simulink model "simulation_main"  (R2025b)
settings: Solver=FixedStepAuto  StartTime=0.0  StopTime=40  RelTol=1e-3
StartFcn:
  | MaxMissedTicks = 99^100;
  | SampleTime = 0.01;
libraries: simulink x5, SignalEditorBlockLib x3
settings Model: Creator=labadmin  LastModifiedBy=David
settings HardwareCC: ProdBitPerLong=64.0  ProdHWDeviceType=Intel->x86-64 (Linux 64)
settings RTWCC: SystemTargetFile=sldrt.tlc  TemplateMakefile=sldrt.tmf  RTWCompilerOptimization=on  GPUComputeCapability=3.5  Description=Simulink Desktop Real-Time
settings CodeAppCC: MaxIdLength=95.0
settings SimulinkDesktopRealTimeCC: ExtModeTransport=0.0  ExtModeStaticAllocSize=1000000.0  TargetLibSuffix=_sldrt.a  TargetPreCompLibLocation=C:\Program Files\MATLAB\R2025b\toolbox\sldrt\lib\win64  MultiwordLength=2048.0  DynamicStringBufferSize=256.0  ParMdlRefBuildCompliant=on  PreserveMATLABNamespacesInGeneratedCode=on  SubcomponentCodeInterfacePackaging=Reusable function

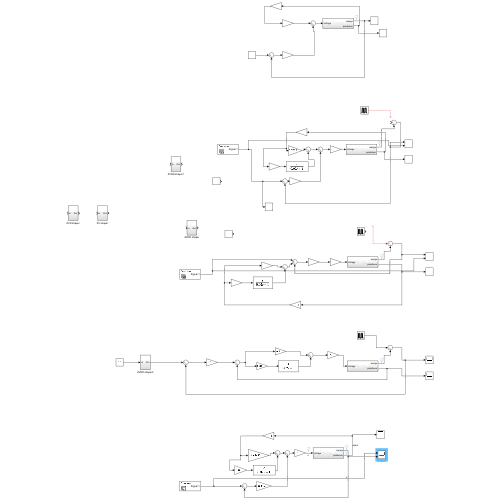
[thumbnail: Simulink's stored preview of the top-level diagram]
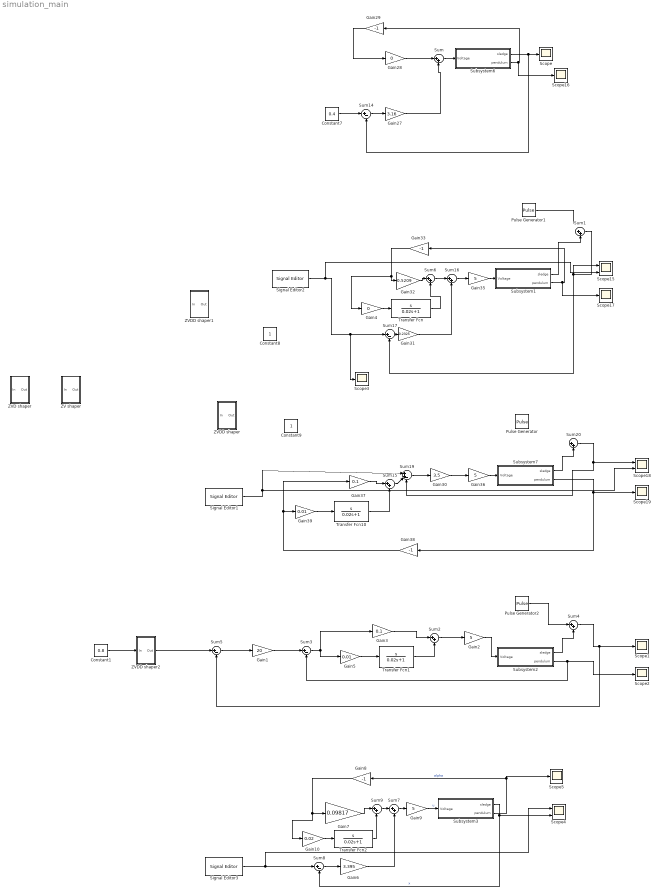
== system simulation_main ==
  Constant1 : Constant  Value=0.8
  Constant7 : Constant  Value=0.4
  Constant8 : Constant
  Constant9 : Constant
  Gain1 : Gain  Gain=20
  Gain10 : Gain  Gain=0.02
  Gain{2,9,35..36} (4 alike) : Gain  Gain=5
  Gain27 : Gain  Gain=3.16
  Gain28 : Gain  Gain=0
  Gain{8,29,33,38} (4 alike) : Gain  Gain=-1
  Gain3 : Gain  Gain=0.1
  Gain30 : Gain  Gain=3.5
  Gain31 : Gain  Gain=0.2325
  Gain32 : Gain  Gain=0.5209
  Gain37 : Gain  Gain=0.1
  Gain39 : Gain  Gain=0.01
  Gain4 : Gain  Gain=0
  Gain5 : Gain  Gain=0.01
  Gain6 : Gain  Gain=3.395
  Gain7 : Gain  Gain=0.09817
  Pulse Generator : DiscretePulseGenerator  PulseType=Time based  Amplitude=0.3  Period=10  PulseWidth=5  PhaseDelay=8
  Pulse Generator1 : DiscretePulseGenerator  PulseType=Time based  Amplitude=0.3  Period=10  PulseWidth=5  PhaseDelay=8
  Pulse Generator2 : DiscretePulseGenerator  PulseType=Time based  Amplitude=0.3  Period=10  PulseWidth=5  PhaseDelay=8
  Scope{,1..3,5,16..17,19} (8 alike) : Scope
      Scope settings: ActiveDisplayYMinimum=-1  ActiveDisplayYMaximum=1  DataLoggingVariableName=ScopeData14
      Scope1 settings: ActiveDisplayYMinimum=-0.13742732109058103  ActiveDisplayYMaximum=1.2368458898152295
      Scope16 settings: ActiveDisplayYMinimum=-1  ActiveDisplayYMaximum=1  DataLoggingVariableName=ScopeData16
      Scope17 settings: ActiveDisplayYMinimum=-3.2028310093193864  ActiveDisplayYMaximum=3.1417469942521352  DataLoggingVariableName=ScopeData17
      Scope19 settings: ActiveDisplayYMinimum=-3.7140586627539296  ActiveDisplayYMaximum=6.2958701074379677  DataLoggingVariableName=ScopeData19
      Scope2 settings: ActiveDisplayYMinimum=-4.882483698452984  ActiveDisplayYMaximum=5.8419143490510415
      Scope3 settings: ActiveDisplayYMinimum=-0.13747885625861364  ActiveDisplayYMaximum=1.2373097063275229  DataLoggingVariableName=ScopeData2
      Scope5 settings: ActiveDisplayYMinimum=-7.2420396350366971  ActiveDisplayYMaximum=11.998274081156339  DataLoggingVariableName=ScopeData4
  Scope15 : Scope  NumInputPorts=2
      settings: ActiveDisplayYMinimum=-0.10013893848214284  ActiveDisplayYMaximum=0.90001543760912706  DataLoggingVariableName=ScopeData15
  Scope18 : Scope  NumInputPorts=2
      settings: ActiveDisplayYMinimum=-1  ActiveDisplayYMaximum=1  DataLoggingVariableName=ScopeData18
  Scope4 : Scope  NumInputPorts=2
      settings: ActiveDisplayYMinimum=-0.10015884989081418  ActiveDisplayYMaximum=0.90005454950171959  DataLoggingVariableName=ScopeData3
  Signal Editor1 : SignalEditorBlockLib/Signal Editor  FileName=input_tuning.mat  ActiveScenario=Scenario  ActiveSignal=Signal 1  IsBus=off  OutputBusObjectStr=Bus: BusObject  SampleTime=0  ZeroCross=off  OutputAfterFinalValue=Setting to zero  Unit=inherit  PreserveSignalName=on  ApplySigPropsToAllScenarios=on  ApplySigPropsToAllSignals=off  SignalPropertySource=Dialog parameters
  Signal Editor2 : SignalEditorBlockLib/Signal Editor  FileName=input_tuning.mat  ActiveScenario=Scenario  ActiveSignal=Signal 1  IsBus=off  OutputBusObjectStr=Bus: BusObject  SampleTime=0  ZeroCross=off  OutputAfterFinalValue=Setting to zero  Unit=inherit  PreserveSignalName=on  ApplySigPropsToAllScenarios=on  ApplySigPropsToAllSignals=off  SignalPropertySource=Dialog parameters
  Signal Editor3 : SignalEditorBlockLib/Signal Editor  FileName=input_tuning.mat  ActiveScenario=Scenario  ActiveSignal=Signal 1  IsBus=off  OutputBusObjectStr=Bus: BusObject  SampleTime=0  ZeroCross=off  OutputAfterFinalValue=Setting to zero  Unit=inherit  PreserveSignalName=on  ApplySigPropsToAllScenarios=on  ApplySigPropsToAllSignals=off  SignalPropertySource=Dialog parameters
  Subsystem1 : Subsystem
  Subsystem2 : Subsystem
  Subsystem3 : Subsystem
  Subsystem6 : Subsystem
  Subsystem7 : Subsystem
  Sum{,1..2,4,6..7,9,15..16,20} (10 alike) : Sum  Inputs=|++
  Sum{3,5,8,14,17} (5 alike) : Sum  Inputs=|+-
  Sum19 : Sum  Inputs=|++-
  Transfer Fcn{,1..2,10} (4 alike) : TransferFcn  Numerator=[1 0]  Denominator=[0.02 1]
  ZV shaper : Subsystem
  ZVD shaper : Subsystem
  ZVDD shaper : Subsystem
  ZVDD shaper1 : Subsystem
  ZVDD shaper2 : Subsystem
  wires:
  Subsystem6/1(sledge) -> Sum14/2, Scope/1
  Sum/1 -> Subsystem6/1(Voltage)
  Constant7/1 -> Sum14/1
  Gain28/1 -> Sum/1
  Subsystem6/2(pendulum) -> Scope16/1, Gain29/1
  Sum14/1 -> Gain27/1
  Gain29/1 -> Gain28/1
  Gain27/1 -> Sum/2
  Gain31/1 -> Sum16/2
  Gain33/1 -> Gain4/1, Gain32/1
  Sum17/1 -> Gain31/1
  Subsystem1/2(pendulum) -> Gain33/1, Scope17/1
  Gain32/1 -> Sum6/1
  Sum16/1 -> Gain35/1
  Sum1/1 -> Scope15/1, Sum17/2
  Gain35/1 -> Subsystem1/1(Voltage)
  Signal Editor2/1 -> Scope15/2, Scope3/1, Sum17/1
  Gain30/1 -> Gain36/1
  Sum19/1 -> Gain30/1
  Gain36/1 -> Subsystem7/1(Voltage)
  Sum20/1 -> Sum19/3, Scope18/1
  Subsystem7/2(pendulum) -> Scope19/1, Gain38/1
  Gain37/1 -> Sum15/1
  Gain38/1 -> Gain39/1, Gain37/1
  Sum15/1 -> Sum19/2
  Transfer Fcn10/1 -> Sum15/2
  Gain39/1 -> Transfer Fcn10/1
  Signal Editor1/1 -> Sum19/1, Scope18/2
  Subsystem7/1(sledge) -> Sum20/2
  ? -> Sum20/1
  Pulse Generator1/1 -> ?
  Subsystem1/1(sledge) -> Sum1/2
  Sum4/1 -> Sum5/2, Scope1/1
  Pulse Generator2/1 -> Sum4/1
  ZVDD shaper2/1(Out) -> Sum5/1
  Subsystem2/1(sledge) -> Sum4/2
  Constant1/1 -> ZVDD shaper2/1(In)
  Gain2/1 -> Subsystem2/1(Voltage)
  Sum2/1 -> Gain2/1
  Gain5/1 -> Transfer Fcn1/1
  Sum3/1 -> Gain3/1, Gain5/1
  Gain3/1 -> Sum2/1
  Transfer Fcn1/1 -> Sum2/2
  Subsystem2/2(pendulum) -> Sum3/2, Scope2/1
  Sum5/1 -> Gain1/1
  Gain1/1 -> Sum3/1
  Transfer Fcn/1 -> Sum6/2
  Gain4/1 -> Transfer Fcn/1
  Sum6/1 -> Sum16/1
  Sum8/1 -> Gain6/1
  Gain8/1 -> Gain10/1, Gain7/1
  Gain7/1 -> Sum9/1
  Gain6/1 -> Sum7/2
  Sum9/1 -> Sum7/1
  Gain10/1 -> Transfer Fcn2/1
  Subsystem3/1(sledge) -> Sum8/2, Scope4/2  "x"
  Transfer Fcn2/1 -> Sum9/2
  Gain9/1 -> Subsystem3/1(Voltage)  "u"
  Subsystem3/2(pendulum) -> Gain8/1, Scope5/1  "alpha"
  Sum7/1 -> Gain9/1
  Signal Editor3/1 -> Scope4/1, Sum8/1

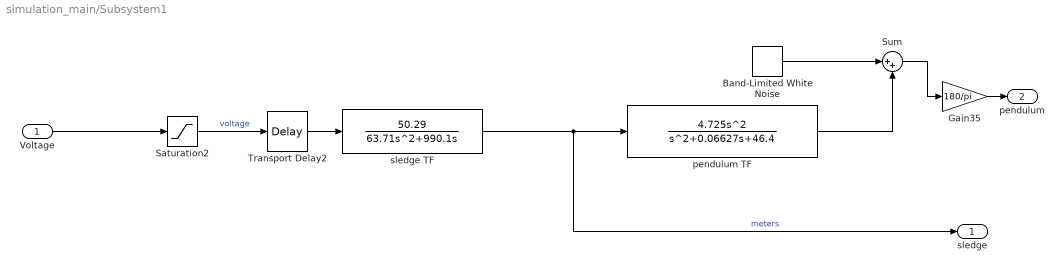
== system simulation_main/Subsystem1 ==
  Voltage : Inport
  Band-Limited White Noise : simulink/Sources/Band-Limited White Noise  Cov=[6e-09]  Ts=0.01  seed=[23341]
  Gain35 : Gain  Gain=180/pi
  Saturation2 : Saturate  UpperLimit=12  LowerLimit=-12
  Sum : Sum  Inputs=|++
  Transport Delay2 : TransportDelay  DelayTime=0.01
  pendulum TF : TransferFcn  Numerator=[4.725 0 0]  Denominator=[1 0.06627 46.4]
  sledge TF : TransferFcn  Numerator=50.29  Denominator="[63.71  990.1 0]"
  sledge : Outport
  pendulum : Outport  Port=2
  wires:
  Saturation2/1 -> Transport Delay2/1  "voltage"
  sledge TF/1 -> pendulum TF/1, sledge/1  "meters"
  Band-Limited White Noise/1 -> Sum/1
  Sum/1 -> Gain35/1
  Voltage/1 -> Saturation2/1
  Transport Delay2/1 -> sledge TF/1
  pendulum TF/1 -> Sum/2
  Gain35/1 -> pendulum/1

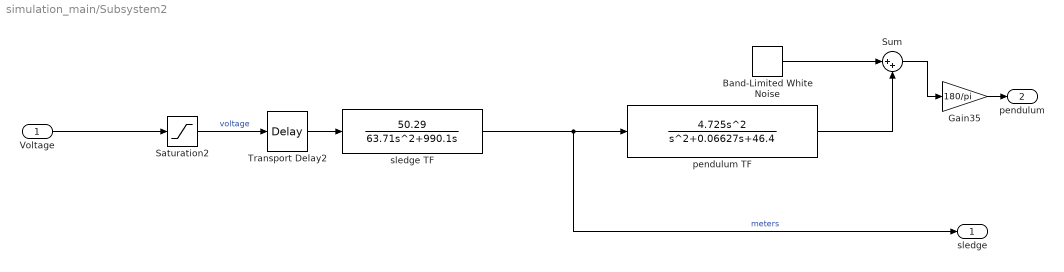
== system simulation_main/Subsystem2 ==
  Voltage : Inport
  Band-Limited White Noise : simulink/Sources/Band-Limited White Noise  Cov=[6e-09]  Ts=0.01  seed=[23341]
  Gain35 : Gain  Gain=180/pi
  Saturation2 : Saturate  UpperLimit=12  LowerLimit=-12
  Sum : Sum  Inputs=|++
  Transport Delay2 : TransportDelay  DelayTime=0.01
  pendulum TF : TransferFcn  Numerator=[4.725 0 0]  Denominator=[1 0.06627 46.4]
  sledge TF : TransferFcn  Numerator=50.29  Denominator="[63.71  990.1 0]"
  sledge : Outport
  pendulum : Outport  Port=2
  wires:
  Saturation2/1 -> Transport Delay2/1  "voltage"
  sledge TF/1 -> pendulum TF/1, sledge/1  "meters"
  Band-Limited White Noise/1 -> Sum/1
  Sum/1 -> Gain35/1
  Voltage/1 -> Saturation2/1
  Transport Delay2/1 -> sledge TF/1
  pendulum TF/1 -> Sum/2
  Gain35/1 -> pendulum/1

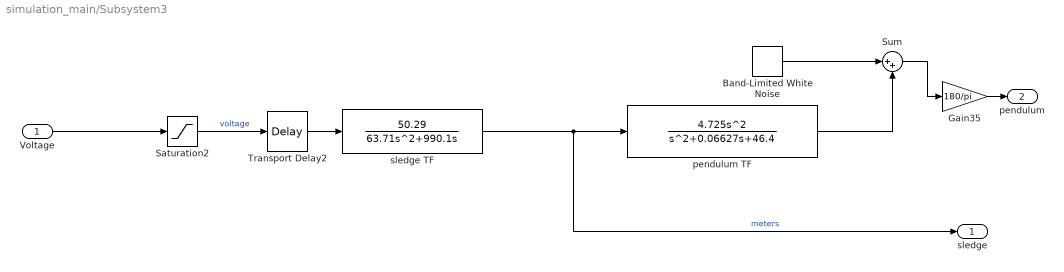
== system simulation_main/Subsystem3 ==
  Voltage : Inport
  Band-Limited White Noise : simulink/Sources/Band-Limited White Noise  Cov=[6e-09]  Ts=0.01  seed=[23341]
  Gain35 : Gain  Gain=180/pi
  Saturation2 : Saturate  UpperLimit=12  LowerLimit=-12
  Sum : Sum  Inputs=|++
  Transport Delay2 : TransportDelay  DelayTime=0.01
  pendulum TF : TransferFcn  Numerator=[4.725 0 0]  Denominator=[1 0.06627 46.4]
  sledge TF : TransferFcn  Numerator=50.29  Denominator="[63.71  990.1 0]"
  sledge : Outport
  pendulum : Outport  Port=2
  wires:
  Saturation2/1 -> Transport Delay2/1  "voltage"
  sledge TF/1 -> pendulum TF/1, sledge/1  "meters"
  Band-Limited White Noise/1 -> Sum/1
  Sum/1 -> Gain35/1
  Voltage/1 -> Saturation2/1
  Transport Delay2/1 -> sledge TF/1
  pendulum TF/1 -> Sum/2
  Gain35/1 -> pendulum/1

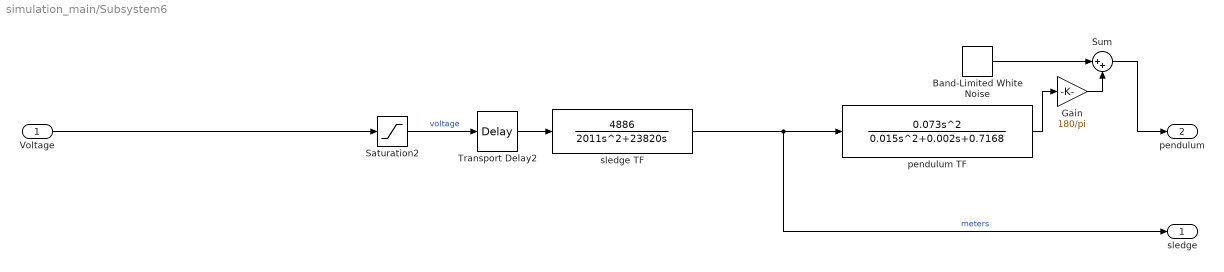
== system simulation_main/Subsystem6 ==
  Voltage : Inport
  Band-Limited White Noise : simulink/Sources/Band-Limited White Noise  Cov=[4.9008e-09]  Ts=0.01  seed=[23341]
  Gain : Gain  Gain=180/pi
  Saturation2 : Saturate  UpperLimit=12  LowerLimit=-12
  Sum : Sum  Inputs=|++
  Transport Delay2 : TransportDelay  DelayTime=0.01
  pendulum TF : TransferFcn  Numerator=[0.073 0 0]  Denominator=[0.015 0.002 0.7168]
  sledge TF : TransferFcn  Numerator=4886  Denominator=[2011 23820 0]
  sledge : Outport
  pendulum : Outport  Port=2
  wires:
  Saturation2/1 -> Transport Delay2/1  "voltage"
  sledge TF/1 -> pendulum TF/1, sledge/1  "meters"
  pendulum TF/1 -> Gain/1
  Band-Limited White Noise/1 -> Sum/1
  Sum/1 -> pendulum/1
  Voltage/1 -> Saturation2/1
  Transport Delay2/1 -> sledge TF/1
  Gain/1 -> Sum/2

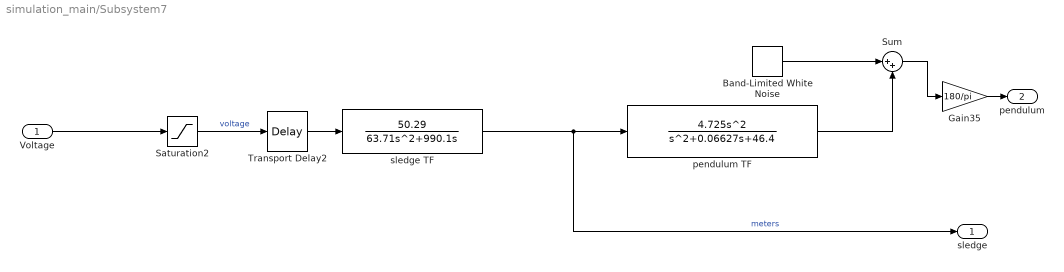
== system simulation_main/Subsystem7 ==
  Voltage : Inport
  Band-Limited White Noise : simulink/Sources/Band-Limited White Noise  Cov=[6e-09]  Ts=0.01  seed=[23341]
  Gain35 : Gain  Gain=180/pi
  Saturation2 : Saturate  UpperLimit=12  LowerLimit=-12
  Sum : Sum  Inputs=|++
  Transport Delay2 : TransportDelay  DelayTime=0.01
  pendulum TF : TransferFcn  Numerator=[4.725 0 0]  Denominator=[1 0.06627 46.4]
  sledge TF : TransferFcn  Numerator=50.29  Denominator="[63.71  990.1 0]"
  sledge : Outport
  pendulum : Outport  Port=2
  wires:
  Saturation2/1 -> Transport Delay2/1  "voltage"
  sledge TF/1 -> pendulum TF/1, sledge/1  "meters"
  Band-Limited White Noise/1 -> Sum/1
  Sum/1 -> Gain35/1
  Voltage/1 -> Saturation2/1
  Transport Delay2/1 -> sledge TF/1
  pendulum TF/1 -> Sum/2
  Gain35/1 -> pendulum/1

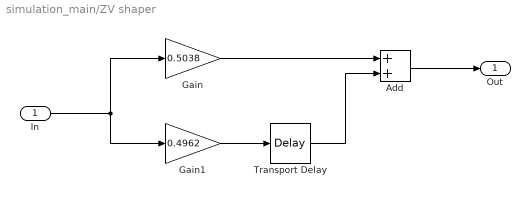
== system simulation_main/ZV shaper ==
  In : Inport
  Add : Sum
  Gain : Gain  Gain=0.5038
  Gain1 : Gain  Gain=0.4962
  Transport Delay : TransportDelay  DelayTime=0.4612
  Out : Outport
  wires:
  Add/1 -> Out/1
  In/1 -> Gain/1, Gain1/1
  Gain1/1 -> Transport Delay/1
  Transport Delay/1 -> Add/2
  Gain/1 -> Add/1

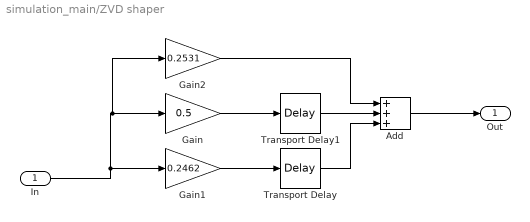
== system simulation_main/ZVD shaper ==
  In : Inport
  Add : Sum  Inputs=+++
  Gain : Gain  Gain=0.5
  Gain1 : Gain  Gain=0.2462
  Gain2 : Gain  Gain=0.2531
  Transport Delay : TransportDelay  DelayTime=0.9224
  Transport Delay1 : TransportDelay  DelayTime=0.4607
  Out : Outport
  wires:
  Gain/1 -> Transport Delay1/1
  Gain1/1 -> Transport Delay/1
  In/1 -> Gain1/1, Gain2/1, Gain/1
  Add/1 -> Out/1
  Transport Delay1/1 -> Add/2
  Transport Delay/1 -> Add/3
  Gain2/1 -> Add/1

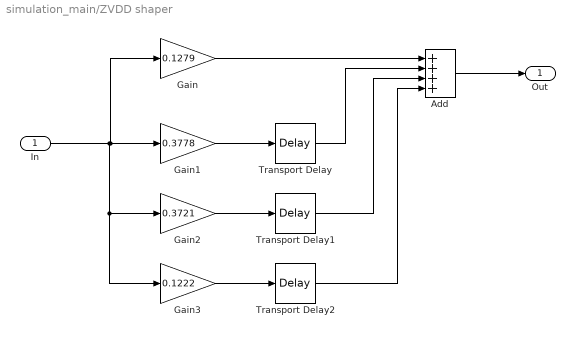
== system simulation_main/ZVDD shaper ==
  In : Inport
  Add : Sum  Inputs=++++
  Gain : Gain  Gain=0.1279
  Gain1 : Gain  Gain=0.3778
  Gain2 : Gain  Gain=0.3721
  Gain3 : Gain  Gain=0.1222
  Transport Delay : TransportDelay  DelayTime=0.4612
  Transport Delay1 : TransportDelay  DelayTime=0.9224
  Transport Delay2 : TransportDelay  DelayTime=1.3836
  Out : Outport
  wires:
  Add/1 -> Out/1
  In/1 -> Gain/1, Gain1/1, Gain3/1, Gain2/1
  Gain1/1 -> Transport Delay/1
  Transport Delay/1 -> Add/2
  Gain/1 -> Add/1
  Gain3/1 -> Transport Delay2/1
  Gain2/1 -> Transport Delay1/1
  Transport Delay1/1 -> Add/3
  Transport Delay2/1 -> Add/4

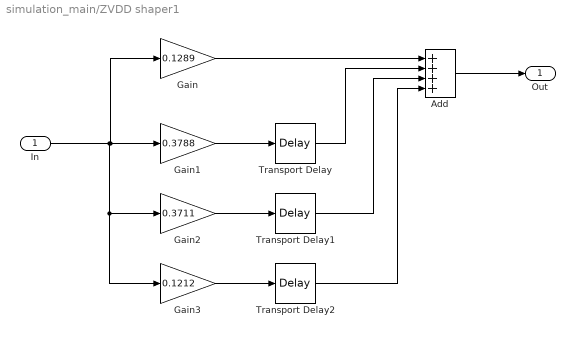
== system simulation_main/ZVDD shaper1 ==
  In : Inport
  Add : Sum  Inputs=++++
  Gain : Gain  Gain=0.1289
  Gain1 : Gain  Gain=0.3788
  Gain2 : Gain  Gain=0.3711
  Gain3 : Gain  Gain=0.1212
  Transport Delay : TransportDelay  DelayTime=0.4607
  Transport Delay1 : TransportDelay  DelayTime=0.9215
  Transport Delay2 : TransportDelay  DelayTime=1.3822
  Out : Outport
  wires:
  Add/1 -> Out/1
  In/1 -> Gain/1, Gain1/1, Gain3/1, Gain2/1
  Gain1/1 -> Transport Delay/1
  Transport Delay/1 -> Add/2
  Gain/1 -> Add/1
  Gain3/1 -> Transport Delay2/1
  Gain2/1 -> Transport Delay1/1
  Transport Delay1/1 -> Add/3
  Transport Delay2/1 -> Add/4

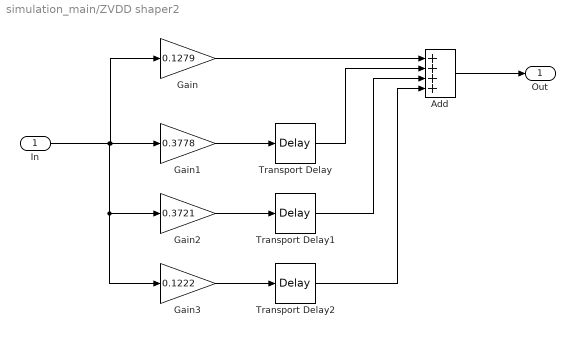
== system simulation_main/ZVDD shaper2 ==
  In : Inport
  Add : Sum  Inputs=++++
  Gain : Gain  Gain=0.1279
  Gain1 : Gain  Gain=0.3778
  Gain2 : Gain  Gain=0.3721
  Gain3 : Gain  Gain=0.1222
  Transport Delay : TransportDelay  DelayTime=0.4612
  Transport Delay1 : TransportDelay  DelayTime=0.9224
  Transport Delay2 : TransportDelay  DelayTime=1.3836
  Out : Outport
  wires:
  Add/1 -> Out/1
  In/1 -> Gain/1, Gain1/1, Gain3/1, Gain2/1
  Gain1/1 -> Transport Delay/1
  Transport Delay/1 -> Add/2
  Gain/1 -> Add/1
  Gain3/1 -> Transport Delay2/1
  Gain2/1 -> Transport Delay1/1
  Transport Delay1/1 -> Add/3
  Transport Delay2/1 -> Add/4
